simulink model "platafomra_esfera"  (R2018b)
settings: Solver=FixedStepAuto  StartTime=0.0  StopTime=30  FixedStep=0.001  RelTol=1e-4
model workspace: external: MATLAB File C:\Users\yomer\OneDrive\MATLAB\tesis\simulacion\platafomra_esfera_DataFile.m (data not in the file)
undefined symbols (not defined in the file or in its folder): a, B, b, HPrd, HPrn, HPtd, HPtn, LPd, LPn, P, rate_lim, smiData, X, Y, Z, z
libraries: sm_lib x73, nesl_utility x19, simulink x3
(part 3 of 3)

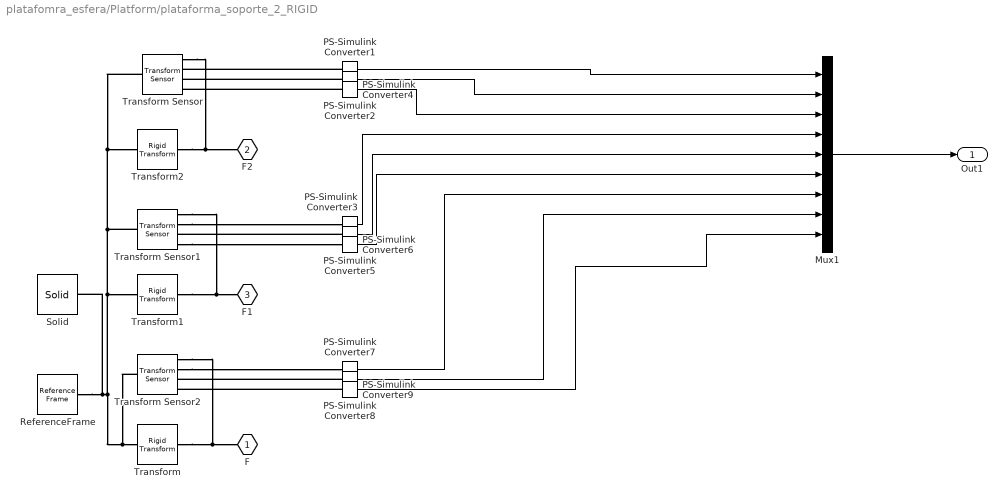
== system platafomra_esfera/Platform/plataforma_soporte_2_RIGID ==
  Mux1 : Mux  Inputs=9
  PS-Simulink Converter{1..9} (9 alike) : nesl_utility/PS-Simulink Converter  PhysicalDomain=network_engine_domain  SubClassName=ps_output  LeftPortType=input  RightPortType=output  PseudoPeriodic=off  Frequencies=[]  Unit=1  AffineConversion=off
  ReferenceFrame : sm_lib/Frames and Transforms/Reference Frame
  Solid : sm_lib/Body Elements/Solid  InertiaType=Custom  Mass=smiData.Solid(7).mass  MassUnits=kg  CenterOfMass=smiData.Solid(7).CoM  CenterOfMassUnits=mm  MomentsOfInertia=smiData.Solid(7).MoI  MomentsOfInertiaUnits=kg*mm^2  ProductsOfInertia=smiData.Solid(7).PoI  ProductsOfInertiaUnits=kg*mm^2  BasedOnType=Density  Density=1000  DensityUnits=kg/m^3  DoExposeReferenceFrame=on  SerializedFrames=<Frames/>  GraphicType=FromGeometry  MarkerShape=Sphere  MarkerSize=10  GraphicVisPropType=SimpleVisualProperties  GraphicDiffuseColor=smiData.Solid(7).color  GraphicSpecularColor=[0.5 0.5 0.5 1.0]  GraphicAmbientColor=[0.15 0.15 0.15 1.0]  GraphicEmissiveColor=[0.0 0.0 0.0 1.0]  GraphicShininess=75  GraphicOpacity=smiData.Solid(7).opacity  GeometryShape=FromFile  RectangleSize=[1 1]  RectangleSizeUnits=m  BrickDimensions=[1 1 1]  BrickDimensionUnits=m  CylinderRadius=1  CylinderRadiusUnits=m  CylinderLength=1  CylinderLengthUnits=m  SphereRadius=1  SphereRadiusUnits=m  EllipsoidRadii=[1 1 1]  EllipsoidRadiiUnits=m  ExtrusionCrossSection=[1 1; -1 1; -1 -1; 1 -1]  ExtrusionCrossSectionUnits=m  ExtrusionLength=1  ExtrusionLengthUnits=m  PolygonNumSides=3  PolygonOuterRadius=1  PolygonOuterRadiusUnits=m  ExtGeomFileType=STEP  ExtGeomFileName=plataforma_soporte_Predeterminado_sldprt.STEP  ExtGeomFileUnits=m  RevolutionCrossSection=[1 1; 1 -1; 2 -1; 2 1]  RevolutionCrossSectionUnits=m  RevolutionExtent=Full  RevolutionAngle=180  RevolutionAngleUnits=deg
  Transform : sm_lib/Frames and Transforms/Rigid Transform  TranslationMethod=Cartesian  TranslationStandardOffset=0  TranslationLengthUnit=mm  TranslationStandardAxis=+Z  TranslationCartesianOffset=smiData.RigidTransform(14).translation  TranslationROffset=0  TranslationROffsetUnits=m  TranslationZOffset=0  TranslationZOffsetUnits=m  TranslationThetaOffset=0  TranslationThetaOffsetUnits=deg  RotationMethod=ArbitraryAxis  RotationAngleUnits=rad  RotationStandardAxis=+Z  RotationAngle=smiData.RigidTransform(14).angle  RotationArbitraryAxis=smiData.RigidTransform(14).axis  FollAlignAxisA=+X  BaseAlignAxisA=+Y  FollAlignAxisB=+Y  BaseAlignAxisB=+Z  RotationSequenceAxes=FollowerAxes  RotationSequence=XYX  RotationSequenceAngles=[0 0 0]  RotationSequenceAnglesUnits=deg  RotationMatrix=[1 0 0; 0 1 0; 0 0 1]
  Transform Sensor : sm_lib/Frames and Transforms/Transform Sensor  MeasurementFrame=World  SenseAngle=off  SenseAxis=off  SenseAngle1=off  SenseAngle2=off  SenseAngle3=off  SenseQ=off  SenseR=off  SenseOmegaX=off  SenseOmegaY=off  SenseOmegaZ=off  SenseOmega1=off  SenseOmega2=off  SenseOmega3=off  SenseQDot=off  SenseRDot=off  SenseAlphaX=off  SenseAlphaY=off  SenseAlphaZ=off  SenseAlpha1=off  SenseAlpha2=off  SenseAlpha3=off  SenseQDDot=off  SenseRDDot=off  SenseX=on  SenseY=on  SenseZ=on  SenseRad=off  SenseAzim=off  SenseDist=off  SenseInc=off  SenseXDot=off  SenseYDot=off  SenseZDot=off  SenseRadDot=off  SenseAzimDot=off  SenseDistDot=off  SenseIncDot=off  SenseXDDot=off  SenseYDDot=off  SenseZDDot=off  SenseRadDDot=off  SenseAzimDDot=off  SenseDistDDot=off  SenseIncDDot=off
  Transform Sensor1 : sm_lib/Frames and Transforms/Transform Sensor  MeasurementFrame=World  SenseAngle=off  SenseAxis=off  SenseAngle1=off  SenseAngle2=off  SenseAngle3=off  SenseQ=off  SenseR=off  SenseOmegaX=off  SenseOmegaY=off  SenseOmegaZ=off  SenseOmega1=off  SenseOmega2=off  SenseOmega3=off  SenseQDot=off  SenseRDot=off  SenseAlphaX=off  SenseAlphaY=off  SenseAlphaZ=off  SenseAlpha1=off  SenseAlpha2=off  SenseAlpha3=off  SenseQDDot=off  SenseRDDot=off  SenseX=on  SenseY=on  SenseZ=on  SenseRad=off  SenseAzim=off  SenseDist=off  SenseInc=off  SenseXDot=off  SenseYDot=off  SenseZDot=off  SenseRadDot=off  SenseAzimDot=off  SenseDistDot=off  SenseIncDot=off  SenseXDDot=off  SenseYDDot=off  SenseZDDot=off  SenseRadDDot=off  SenseAzimDDot=off  SenseDistDDot=off  SenseIncDDot=off
  Transform Sensor2 : sm_lib/Frames and Transforms/Transform Sensor  MeasurementFrame=World  SenseAngle=off  SenseAxis=off  SenseAngle1=off  SenseAngle2=off  SenseAngle3=off  SenseQ=off  SenseR=off  SenseOmegaX=off  SenseOmegaY=off  SenseOmegaZ=off  SenseOmega1=off  SenseOmega2=off  SenseOmega3=off  SenseQDot=off  SenseRDot=off  SenseAlphaX=off  SenseAlphaY=off  SenseAlphaZ=off  SenseAlpha1=off  SenseAlpha2=off  SenseAlpha3=off  SenseQDDot=off  SenseRDDot=off  SenseX=on  SenseY=on  SenseZ=on  SenseRad=off  SenseAzim=off  SenseDist=off  SenseInc=off  SenseXDot=off  SenseYDot=off  SenseZDot=off  SenseRadDot=off  SenseAzimDot=off  SenseDistDot=off  SenseIncDot=off  SenseXDDot=off  SenseYDDot=off  SenseZDDot=off  SenseRadDDot=off  SenseAzimDDot=off  SenseDistDDot=off  SenseIncDDot=off
  Transform1 : sm_lib/Frames and Transforms/Rigid Transform  TranslationMethod=Cartesian  TranslationStandardOffset=0  TranslationLengthUnit=mm  TranslationStandardAxis=+Z  TranslationCartesianOffset=smiData.RigidTransform(16).translation  TranslationROffset=0  TranslationROffsetUnits=m  TranslationZOffset=0  TranslationZOffsetUnits=m  TranslationThetaOffset=0  TranslationThetaOffsetUnits=deg  RotationMethod=ArbitraryAxis  RotationAngleUnits=rad  RotationStandardAxis=+Z  RotationAngle=smiData.RigidTransform(16).angle  RotationArbitraryAxis=smiData.RigidTransform(16).axis  FollAlignAxisA=+X  BaseAlignAxisA=+Y  FollAlignAxisB=+Y  BaseAlignAxisB=+Z  RotationSequenceAxes=FollowerAxes  RotationSequence=XYX  RotationSequenceAngles=[0 0 0]  RotationSequenceAnglesUnits=deg  RotationMatrix=[1 0 0; 0 1 0; 0 0 1]
  Transform2 : sm_lib/Frames and Transforms/Rigid Transform  TranslationMethod=Cartesian  TranslationStandardOffset=0  TranslationLengthUnit=mm  TranslationStandardAxis=+Z  TranslationCartesianOffset=smiData.RigidTransform(18).translation  TranslationROffset=0  TranslationROffsetUnits=m  TranslationZOffset=0  TranslationZOffsetUnits=m  TranslationThetaOffset=0  TranslationThetaOffsetUnits=deg  RotationMethod=ArbitraryAxis  RotationAngleUnits=rad  RotationStandardAxis=+Z  RotationAngle=smiData.RigidTransform(18).angle  RotationArbitraryAxis=smiData.RigidTransform(18).axis  FollAlignAxisA=+X  BaseAlignAxisA=+Y  FollAlignAxisB=+Y  BaseAlignAxisB=+Z  RotationSequenceAxes=FollowerAxes  RotationSequence=XYX  RotationSequenceAngles=[0 0 0]  RotationSequenceAnglesUnits=deg  RotationMatrix=[1 0 0; 0 1 0; 0 0 1]
  F : PMIOPort  Side=Left
  F2 : PMIOPort  Port=2  Side=Left
  F1 : PMIOPort  Port=3  Side=Left
  Out1 : Outport
  wires:
  PS-Simulink Converter5/1 -> Mux1/5
  PS-Simulink Converter8/1 -> Mux1/8
  PS-Simulink Converter3/1 -> Mux1/4
  PS-Simulink Converter6/1 -> Mux1/6
  PS-Simulink Converter7/1 -> Mux1/7
  PS-Simulink Converter9/1 -> Mux1/9
  PS-Simulink Converter4/1 -> Mux1/3
  PS-Simulink Converter1/1 -> Mux1/1
  PS-Simulink Converter2/1 -> Mux1/2
  Mux1/1 -> Out1/1
  connections:
  Solid/RConn1 -- ReferenceFrame/RConn1 -- Transform1/LConn1 -- Transform Sensor/LConn1 -- Transform2/LConn1 -- Transform Sensor1/LConn1 -- Transform Sensor2/LConn1 -- Transform/LConn1
  Transform/RConn1 -- Transform Sensor2/RConn1 -- F/RConn1
  Transform1/RConn1 -- Transform Sensor1/RConn1 -- F1/RConn1
  Transform2/RConn1 -- Transform Sensor/RConn1 -- F2/RConn1
  PS-Simulink Converter1/LConn1 -- Transform Sensor/RConn2
  PS-Simulink Converter2/LConn1 -- Transform Sensor/RConn3
  PS-Simulink Converter4/LConn1 -- Transform Sensor/RConn4
  PS-Simulink Converter9/LConn1 -- Transform Sensor2/RConn4
  PS-Simulink Converter8/LConn1 -- Transform Sensor2/RConn3
  Transform Sensor2/RConn2 -- PS-Simulink Converter7/LConn1
  Transform Sensor1/RConn4 -- PS-Simulink Converter6/LConn1
  PS-Simulink Converter5/LConn1 -- Transform Sensor1/RConn3
  Transform Sensor1/RConn2 -- PS-Simulink Converter3/LConn1

== system platafomra_esfera/Platform/viela2_1_RIGID ==
  ReferenceFrame : sm_lib/Frames and Transforms/Reference Frame
  Solid : sm_lib/Body Elements/Solid  InertiaType=Custom  Mass=smiData.Solid(6).mass  MassUnits=kg  CenterOfMass=smiData.Solid(6).CoM  CenterOfMassUnits=mm  MomentsOfInertia=smiData.Solid(6).MoI  MomentsOfInertiaUnits=kg*mm^2  ProductsOfInertia=smiData.Solid(6).PoI  ProductsOfInertiaUnits=kg*mm^2  BasedOnType=Density  Density=1000  DensityUnits=kg/m^3  DoExposeReferenceFrame=on  SerializedFrames=<Frames/>  GraphicType=FromGeometry  MarkerShape=Sphere  MarkerSize=10  GraphicVisPropType=SimpleVisualProperties  GraphicDiffuseColor=smiData.Solid(6).color  GraphicSpecularColor=[0.5 0.5 0.5 1.0]  GraphicAmbientColor=[0.15 0.15 0.15 1.0]  GraphicEmissiveColor=[0.0 0.0 0.0 1.0]  GraphicShininess=75  GraphicOpacity=smiData.Solid(6).opacity  GeometryShape=FromFile  RectangleSize=[1 1]  RectangleSizeUnits=m  BrickDimensions=[1 1 1]  BrickDimensionUnits=m  CylinderRadius=1  CylinderRadiusUnits=m  CylinderLength=1  CylinderLengthUnits=m  SphereRadius=1  SphereRadiusUnits=m  EllipsoidRadii=[1 1 1]  EllipsoidRadiiUnits=m  ExtrusionCrossSection=[1 1; -1 1; -1 -1; 1 -1]  ExtrusionCrossSectionUnits=m  ExtrusionLength=1  ExtrusionLengthUnits=m  PolygonNumSides=3  PolygonOuterRadius=1  PolygonOuterRadiusUnits=m  ExtGeomFileType=STEP  ExtGeomFileName=viela2_Predeterminado_sldprt.STEP  ExtGeomFileUnits=m  RevolutionCrossSection=[1 1; 1 -1; 2 -1; 2 1]  RevolutionCrossSectionUnits=m  RevolutionExtent=Full  RevolutionAngle=180  RevolutionAngleUnits=deg
  Transform : sm_lib/Frames and Transforms/Rigid Transform  TranslationMethod=Cartesian  TranslationStandardOffset=0  TranslationLengthUnit=mm  TranslationStandardAxis=+Z  TranslationCartesianOffset=smiData.RigidTransform(1).translation  TranslationROffset=0  TranslationROffsetUnits=m  TranslationZOffset=0  TranslationZOffsetUnits=m  TranslationThetaOffset=0  TranslationThetaOffsetUnits=deg  RotationMethod=ArbitraryAxis  RotationAngleUnits=rad  RotationStandardAxis=+Z  RotationAngle=smiData.RigidTransform(1).angle  RotationArbitraryAxis=smiData.RigidTransform(1).axis  FollAlignAxisA=+X  BaseAlignAxisA=+Y  FollAlignAxisB=+Y  BaseAlignAxisB=+Z  RotationSequenceAxes=FollowerAxes  RotationSequence=XYX  RotationSequenceAngles=[0 0 0]  RotationSequenceAnglesUnits=deg  RotationMatrix=[1 0 0; 0 1 0; 0 0 1]
  Transform1 : sm_lib/Frames and Transforms/Rigid Transform  TranslationMethod=Cartesian  TranslationStandardOffset=0  TranslationLengthUnit=mm  TranslationStandardAxis=+Z  TranslationCartesianOffset=smiData.RigidTransform(4).translation  TranslationROffset=0  TranslationROffsetUnits=m  TranslationZOffset=0  TranslationZOffsetUnits=m  TranslationThetaOffset=0  TranslationThetaOffsetUnits=deg  RotationMethod=ArbitraryAxis  RotationAngleUnits=rad  RotationStandardAxis=+Z  RotationAngle=smiData.RigidTransform(4).angle  RotationArbitraryAxis=smiData.RigidTransform(4).axis  FollAlignAxisA=+X  BaseAlignAxisA=+Y  FollAlignAxisB=+Y  BaseAlignAxisB=+Z  RotationSequenceAxes=FollowerAxes  RotationSequence=XYX  RotationSequenceAngles=[0 0 0]  RotationSequenceAnglesUnits=deg  RotationMatrix=[1 0 0; 0 1 0; 0 0 1]
  Transform2 : sm_lib/Frames and Transforms/Rigid Transform  TranslationMethod=Cartesian  TranslationStandardOffset=0  TranslationLengthUnit=mm  TranslationStandardAxis=+Z  TranslationCartesianOffset=smiData.RigidTransform(5).translation  TranslationROffset=0  TranslationROffsetUnits=m  TranslationZOffset=0  TranslationZOffsetUnits=m  TranslationThetaOffset=0  TranslationThetaOffsetUnits=deg  RotationMethod=ArbitraryAxis  RotationAngleUnits=rad  RotationStandardAxis=+Z  RotationAngle=smiData.RigidTransform(5).angle  RotationArbitraryAxis=smiData.RigidTransform(5).axis  FollAlignAxisA=+X  BaseAlignAxisA=+Y  FollAlignAxisB=+Y  BaseAlignAxisB=+Z  RotationSequenceAxes=FollowerAxes  RotationSequence=XYX  RotationSequenceAngles=[0 0 0]  RotationSequenceAnglesUnits=deg  RotationMatrix=[1 0 0; 0 1 0; 0 0 1]
  F1 : PMIOPort  Side=Left
  F2 : PMIOPort  Port=2  Side=Right
  F : PMIOPort  Port=3  Side=Right
  connections:
  Solid/RConn1 -- ReferenceFrame/RConn1 -- Transform/LConn1 -- Transform1/LConn1 -- Transform2/LConn1
  Transform/RConn1 -- F/RConn1
  Transform1/RConn1 -- F1/RConn1
  Transform2/RConn1 -- F2/RConn1

== system platafomra_esfera/Platform/viela3_1_RIGID ==
  ReferenceFrame : sm_lib/Frames and Transforms/Reference Frame
  Solid : sm_lib/Body Elements/Solid  InertiaType=Custom  Mass=smiData.Solid(5).mass  MassUnits=kg  CenterOfMass=smiData.Solid(5).CoM  CenterOfMassUnits=mm  MomentsOfInertia=smiData.Solid(5).MoI  MomentsOfInertiaUnits=kg*mm^2  ProductsOfInertia=smiData.Solid(5).PoI  ProductsOfInertiaUnits=kg*mm^2  BasedOnType=Density  Density=1000  DensityUnits=kg/m^3  DoExposeReferenceFrame=on  SerializedFrames=<Frames/>  GraphicType=FromGeometry  MarkerShape=Sphere  MarkerSize=10  GraphicVisPropType=SimpleVisualProperties  GraphicDiffuseColor=smiData.Solid(5).color  GraphicSpecularColor=[0.5 0.5 0.5 1.0]  GraphicAmbientColor=[0.15 0.15 0.15 1.0]  GraphicEmissiveColor=[0.0 0.0 0.0 1.0]  GraphicShininess=75  GraphicOpacity=smiData.Solid(5).opacity  GeometryShape=FromFile  RectangleSize=[1 1]  RectangleSizeUnits=m  BrickDimensions=[1 1 1]  BrickDimensionUnits=m  CylinderRadius=1  CylinderRadiusUnits=m  CylinderLength=1  CylinderLengthUnits=m  SphereRadius=1  SphereRadiusUnits=m  EllipsoidRadii=[1 1 1]  EllipsoidRadiiUnits=m  ExtrusionCrossSection=[1 1; -1 1; -1 -1; 1 -1]  ExtrusionCrossSectionUnits=m  ExtrusionLength=1  ExtrusionLengthUnits=m  PolygonNumSides=3  PolygonOuterRadius=1  PolygonOuterRadiusUnits=m  ExtGeomFileType=STEP  ExtGeomFileName=viela3_Predeterminado_sldprt.STEP  ExtGeomFileUnits=m  RevolutionCrossSection=[1 1; 1 -1; 2 -1; 2 1]  RevolutionCrossSectionUnits=m  RevolutionExtent=Full  RevolutionAngle=180  RevolutionAngleUnits=deg
  Transform : sm_lib/Frames and Transforms/Rigid Transform  TranslationMethod=Cartesian  TranslationStandardOffset=0  TranslationLengthUnit=mm  TranslationStandardAxis=+Z  TranslationCartesianOffset=smiData.RigidTransform(7).translation  TranslationROffset=0  TranslationROffsetUnits=m  TranslationZOffset=0  TranslationZOffsetUnits=m  TranslationThetaOffset=0  TranslationThetaOffsetUnits=deg  RotationMethod=ArbitraryAxis  RotationAngleUnits=rad  RotationStandardAxis=+Z  RotationAngle=smiData.RigidTransform(7).angle  RotationArbitraryAxis=smiData.RigidTransform(7).axis  FollAlignAxisA=+X  BaseAlignAxisA=+Y  FollAlignAxisB=+Y  BaseAlignAxisB=+Z  RotationSequenceAxes=FollowerAxes  RotationSequence=XYX  RotationSequenceAngles=[0 0 0]  RotationSequenceAnglesUnits=deg  RotationMatrix=[1 0 0; 0 1 0; 0 0 1]
  Transform1 : sm_lib/Frames and Transforms/Rigid Transform  TranslationMethod=Cartesian  TranslationStandardOffset=0  TranslationLengthUnit=mm  TranslationStandardAxis=+Z  TranslationCartesianOffset=smiData.RigidTransform(10).translation  TranslationROffset=0  TranslationROffsetUnits=m  TranslationZOffset=0  TranslationZOffsetUnits=m  TranslationThetaOffset=0  TranslationThetaOffsetUnits=deg  RotationMethod=ArbitraryAxis  RotationAngleUnits=rad  RotationStandardAxis=+Z  RotationAngle=smiData.RigidTransform(10).angle  RotationArbitraryAxis=smiData.RigidTransform(10).axis  FollAlignAxisA=+X  BaseAlignAxisA=+Y  FollAlignAxisB=+Y  BaseAlignAxisB=+Z  RotationSequenceAxes=FollowerAxes  RotationSequence=XYX  RotationSequenceAngles=[0 0 0]  RotationSequenceAnglesUnits=deg  RotationMatrix=[1 0 0; 0 1 0; 0 0 1]
  Transform2 : sm_lib/Frames and Transforms/Rigid Transform  TranslationMethod=Cartesian  TranslationStandardOffset=0  TranslationLengthUnit=mm  TranslationStandardAxis=+Z  TranslationCartesianOffset=smiData.RigidTransform(11).translation  TranslationROffset=0  TranslationROffsetUnits=m  TranslationZOffset=0  TranslationZOffsetUnits=m  TranslationThetaOffset=0  TranslationThetaOffsetUnits=deg  RotationMethod=ArbitraryAxis  RotationAngleUnits=rad  RotationStandardAxis=+Z  RotationAngle=smiData.RigidTransform(11).angle  RotationArbitraryAxis=smiData.RigidTransform(11).axis  FollAlignAxisA=+X  BaseAlignAxisA=+Y  FollAlignAxisB=+Y  BaseAlignAxisB=+Z  RotationSequenceAxes=FollowerAxes  RotationSequence=XYX  RotationSequenceAngles=[0 0 0]  RotationSequenceAnglesUnits=deg  RotationMatrix=[1 0 0; 0 1 0; 0 0 1]
  F1 : PMIOPort  Side=Left
  F2 : PMIOPort  Port=2  Side=Right
  F : PMIOPort  Port=3  Side=Right
  connections:
  Solid/RConn1 -- ReferenceFrame/RConn1 -- Transform/LConn1 -- Transform1/LConn1 -- Transform2/LConn1
  Transform/RConn1 -- F/RConn1
  Transform1/RConn1 -- F1/RConn1
  Transform2/RConn1 -- F2/RConn1

== system platafomra_esfera/Platform/viela_1_RIGID ==
  ReferenceFrame : sm_lib/Frames and Transforms/Reference Frame
  Solid : sm_lib/Body Elements/Solid  InertiaType=Custom  Mass=smiData.Solid(3).mass  MassUnits=kg  CenterOfMass=smiData.Solid(3).CoM  CenterOfMassUnits=mm  MomentsOfInertia=smiData.Solid(3).MoI  MomentsOfInertiaUnits=kg*mm^2  ProductsOfInertia=smiData.Solid(3).PoI  ProductsOfInertiaUnits=kg*mm^2  BasedOnType=Density  Density=1000  DensityUnits=kg/m^3  DoExposeReferenceFrame=on  SerializedFrames=<Frames/>  GraphicType=FromGeometry  MarkerShape=Sphere  MarkerSize=10  GraphicVisPropType=SimpleVisualProperties  GraphicDiffuseColor=smiData.Solid(3).color  GraphicSpecularColor=[0.5 0.5 0.5 1.0]  GraphicAmbientColor=[0.15 0.15 0.15 1.0]  GraphicEmissiveColor=[0.0 0.0 0.0 1.0]  GraphicShininess=75  GraphicOpacity=smiData.Solid(3).opacity  GeometryShape=FromFile  RectangleSize=[1 1]  RectangleSizeUnits=m  BrickDimensions=[1 1 1]  BrickDimensionUnits=m  CylinderRadius=1  CylinderRadiusUnits=m  CylinderLength=1  CylinderLengthUnits=m  SphereRadius=1  SphereRadiusUnits=m  EllipsoidRadii=[1 1 1]  EllipsoidRadiiUnits=m  ExtrusionCrossSection=[1 1; -1 1; -1 -1; 1 -1]  ExtrusionCrossSectionUnits=m  ExtrusionLength=1  ExtrusionLengthUnits=m  PolygonNumSides=3  PolygonOuterRadius=1  PolygonOuterRadiusUnits=m  ExtGeomFileType=STEP  ExtGeomFileName=viela_Predeterminado_sldprt.STEP  ExtGeomFileUnits=m  RevolutionCrossSection=[1 1; 1 -1; 2 -1; 2 1]  RevolutionCrossSectionUnits=m  RevolutionExtent=Full  RevolutionAngle=180  RevolutionAngleUnits=deg
  Transform : sm_lib/Frames and Transforms/Rigid Transform  TranslationMethod=Cartesian  TranslationStandardOffset=0  TranslationLengthUnit=mm  TranslationStandardAxis=+Z  TranslationCartesianOffset=smiData.RigidTransform(25).translation  TranslationROffset=0  TranslationROffsetUnits=m  TranslationZOffset=0  TranslationZOffsetUnits=m  TranslationThetaOffset=0  TranslationThetaOffsetUnits=deg  RotationMethod=ArbitraryAxis  RotationAngleUnits=rad  RotationStandardAxis=+Z  RotationAngle=smiData.RigidTransform(25).angle  RotationArbitraryAxis=smiData.RigidTransform(25).axis  FollAlignAxisA=+X  BaseAlignAxisA=+Y  FollAlignAxisB=+Y  BaseAlignAxisB=+Z  RotationSequenceAxes=FollowerAxes  RotationSequence=XYX  RotationSequenceAngles=[0 0 0]  RotationSequenceAnglesUnits=deg  RotationMatrix=[1 0 0; 0 1 0; 0 0 1]
  Transform1 : sm_lib/Frames and Transforms/Rigid Transform  TranslationMethod=Cartesian  TranslationStandardOffset=0  TranslationLengthUnit=mm  TranslationStandardAxis=+Z  TranslationCartesianOffset=smiData.RigidTransform(28).translation  TranslationROffset=0  TranslationROffsetUnits=m  TranslationZOffset=0  TranslationZOffsetUnits=m  TranslationThetaOffset=0  TranslationThetaOffsetUnits=deg  RotationMethod=ArbitraryAxis  RotationAngleUnits=rad  RotationStandardAxis=+Z  RotationAngle=smiData.RigidTransform(28).angle  RotationArbitraryAxis=smiData.RigidTransform(28).axis  FollAlignAxisA=+X  BaseAlignAxisA=+Y  FollAlignAxisB=+Y  BaseAlignAxisB=+Z  RotationSequenceAxes=FollowerAxes  RotationSequence=XYX  RotationSequenceAngles=[0 0 0]  RotationSequenceAnglesUnits=deg  RotationMatrix=[1 0 0; 0 1 0; 0 0 1]
  Transform2 : sm_lib/Frames and Transforms/Rigid Transform  TranslationMethod=Cartesian  TranslationStandardOffset=0  TranslationLengthUnit=mm  TranslationStandardAxis=+Z  TranslationCartesianOffset=smiData.RigidTransform(29).translation  TranslationROffset=0  TranslationROffsetUnits=m  TranslationZOffset=0  TranslationZOffsetUnits=m  TranslationThetaOffset=0  TranslationThetaOffsetUnits=deg  RotationMethod=ArbitraryAxis  RotationAngleUnits=rad  RotationStandardAxis=+Z  RotationAngle=smiData.RigidTransform(29).angle  RotationArbitraryAxis=smiData.RigidTransform(29).axis  FollAlignAxisA=+X  BaseAlignAxisA=+Y  FollAlignAxisB=+Y  BaseAlignAxisB=+Z  RotationSequenceAxes=FollowerAxes  RotationSequence=XYX  RotationSequenceAngles=[0 0 0]  RotationSequenceAnglesUnits=deg  RotationMatrix=[1 0 0; 0 1 0; 0 0 1]
  F1 : PMIOPort  Side=Left
  F : PMIOPort  Port=2  Side=Right
  F2 : PMIOPort  Port=3  Side=Right
  connections:
  Solid/RConn1 -- ReferenceFrame/RConn1 -- Transform/LConn1 -- Transform1/LConn1 -- Transform2/LConn1
  Transform/RConn1 -- F/RConn1
  Transform1/RConn1 -- F1/RConn1
  Transform2/RConn1 -- F2/RConn1

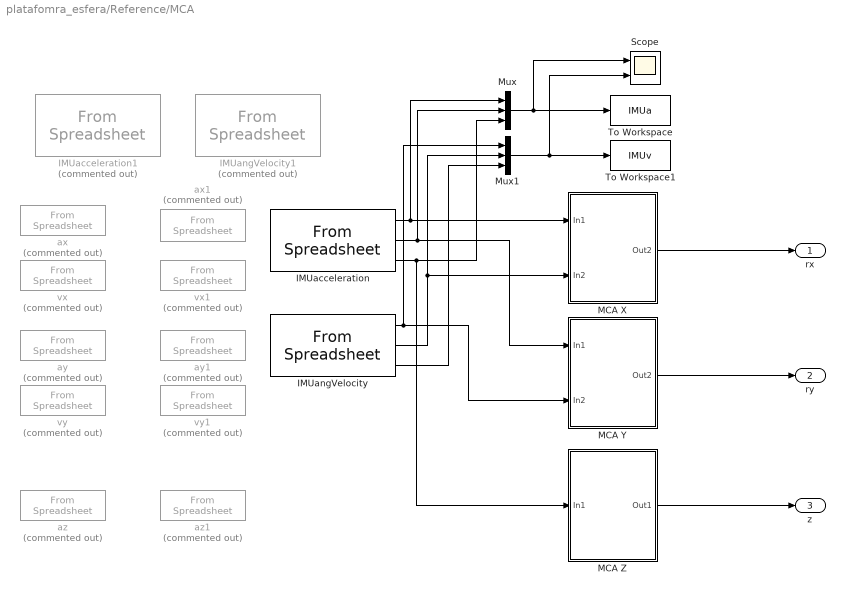
== system platafomra_esfera/Reference/MCA ==
  IMUacceleration : FromSpreadsheet  FileName=arrranqueparo2.xlsx  SheetName=Hoja1  Range=D2:F1014  TreatFirstColumnAs=Data  SampleTime=0.03
  IMUacceleration1 : FromSpreadsheet  Commented=on  FileName=vuelta90deg.xlsx  SheetName=Hoja1  Range=D2:F1089  TreatFirstColumnAs=Data  SampleTime=0.03
  IMUangVelocity : FromSpreadsheet  FileName=arrranqueparo2.xlsx  SheetName=Hoja1  Range=G2:I1014  TreatFirstColumnAs=Data  SampleTime=0.03
  IMUangVelocity1 : FromSpreadsheet  Commented=on  FileName=vuelta90deg.xlsx  SheetName=Hoja1  Range=G2:I1089  TreatFirstColumnAs=Data  SampleTime=0.03
  MCA X : Subsystem
  MCA Y : Subsystem
  MCA Z : Subsystem
  Mux : Mux  Inputs=3
  Mux1 : Mux  Inputs=3
  Scope : Scope  NumInputPorts=2
  To Workspace : ToWorkspace  VariableName=IMUa  SaveFormat=Timeseries  SampleTime=-1
  To Workspace1 : ToWorkspace  VariableName=IMUv  SaveFormat=Timeseries  SampleTime=-1
  ax : FromSpreadsheet  Commented=on  FileName=imu.xlsx  SheetName=Hoja1  Range=A1:A950  TreatFirstColumnAs=Data  SampleTime=0.016
  ax1 : FromSpreadsheet  Commented=on  FileName=arrranqueparo2.xlsx  SheetName=Hoja1  Range=D2:D1014  TreatFirstColumnAs=Data  SampleTime=0.03
  ay : FromSpreadsheet  Commented=on  FileName=imu.xlsx  SheetName=Hoja1  Range=B1:B950  TreatFirstColumnAs=Data  SampleTime=0.016
  ay1 : FromSpreadsheet  Commented=on  FileName=arrranqueparo.xlsx  SheetName=Hoja1  Range=B1:B1028  TreatFirstColumnAs=Data  SampleTime=0.016
  az : FromSpreadsheet  Commented=on  FileName=imu.xlsx  SheetName=Hoja1  Range=C1:C950  TreatFirstColumnAs=Data  SampleTime=0.016
  az1 : FromSpreadsheet  Commented=on  FileName=arrranqueparo.xlsx  SheetName=Hoja1  Range=C1:C1028  TreatFirstColumnAs=Data  SampleTime=0.016
  vx : FromSpreadsheet  Commented=on  FileName=imu.xlsx  SheetName=Hoja1  Range=D1:D950  TreatFirstColumnAs=Data  SampleTime=0.016
  vx1 : FromSpreadsheet  Commented=on  FileName=arrranqueparo.xlsx  SheetName=Hoja1  Range=D1:D1028  TreatFirstColumnAs=Data  SampleTime=0.016
  vy : FromSpreadsheet  Commented=on  FileName=imu.xlsx  SheetName=Hoja1  Range=E1:E950  TreatFirstColumnAs=Data  SampleTime=0.016
  vy1 : FromSpreadsheet  Commented=on  FileName=arrranqueparo.xlsx  SheetName=Hoja1  Range=E1:E1028  TreatFirstColumnAs=Data  SampleTime=0.016
  rx : Outport
  ry : Outport  Port=2
  z : Outport  Port=3
  wires:
  MCA Z/1(Out1) -> z/1
  Mux/1 -> Scope/1, To Workspace/1
  Mux1/1 -> Scope/2, To Workspace1/1
  MCA Y/1(Out2) -> ry/1
  MCA X/1(Out2) -> rx/1
  IMUacceleration/1 -> Mux/1, MCA X/1(In1)
  IMUacceleration/2 -> Mux/2, MCA Y/1(In1)
  IMUacceleration/3 -> Mux/3, MCA Z/1(In1)
  IMUangVelocity/1 -> MCA Y/2(In2), Mux1/1
  IMUangVelocity/2 -> MCA X/2(In2), Mux1/2
  IMUangVelocity/3 -> Mux1/3

== system platafomra_esfera/Reference/Subsystem1 ==
  t : Inport
  Add : Sum  Inputs=|++
  Add2 : Sum  Inputs=++|
  Sin : Trigonometry
  amp1 : Gain  Gain=5
  deg2rad : Gain  Gain=pi/180
  deg2rad2 : Gain  Gain=(pi/180)
  freq : Gain  Gain=360 * 3 / 10
  offset : Constant  Value=0  VectorParams1D=off
  phase : Constant  Value=0  VectorParams1D=off
  f : Outport
  wires:
  t/1 -> freq/1
  Add2/1 -> f/1
  offset/1 -> Add2/1
  freq/1 -> Add/1
  deg2rad/1 -> Sin/1
  Add/1 -> deg2rad/1
  amp1/1 -> deg2rad2/1
  Sin/1 -> amp1/1
  phase/1 -> Add/2
  deg2rad2/1 -> Add2/2

== system platafomra_esfera/Reference/Subsystem3 ==
  t : Inport
  Add : Sum  Inputs=|++
  Add2 : Sum  Inputs=++|
  Sin : Trigonometry
  amp1 : Gain  Gain=5
  deg2rad : Gain  Gain=pi/180
  deg2rad2 : Gain  Gain=(pi/180)
  freq : Gain  Gain=360 * 3 / 10
  offset : Constant  Value=0  VectorParams1D=off
  phase : Constant  Value=-90  VectorParams1D=off
  f : Outport
  wires:
  phase/1 -> Add/2
  Sin/1 -> amp1/1
  amp1/1 -> deg2rad2/1
  Add/1 -> deg2rad/1
  deg2rad/1 -> Sin/1
  freq/1 -> Add/1
  offset/1 -> Add2/1
  Add2/1 -> f/1
  t/1 -> freq/1
  deg2rad2/1 -> Add2/2

== system platafomra_esfera/Reference/Subsystem5 ==
  t : Inport
  Add : Sum  Inputs=|++
  Add2 : Sum  Inputs=++|
  Sin : Trigonometry
  amp1 : Gain  Gain=0.02
  deg2rad : Gain  Gain=pi/180
  freq : Gain  Gain=360 * 5/10
  offset : Constant  Value=0  VectorParams1D=off
  phase : Constant  Value=-90  VectorParams1D=off
  f : Outport
  wires:
  phase/1 -> Add/2
  Sin/1 -> amp1/1
  amp1/1 -> Add2/2
  Add/1 -> deg2rad/1
  deg2rad/1 -> Sin/1
  freq/1 -> Add/1
  offset/1 -> Add2/1
  Add2/1 -> f/1
  t/1 -> freq/1

== system platafomra_esfera/ADRC/Subsystem/ADRC ==
  note: V
  note: u
  x1 : Inport
  x2 : Inport  Port=2
  Z : Inport  Port=3
  xd : Inport  Port=4
  Demux : Demux  Outputs=2
  Derivative1 : Derivative
  MATLAB Function1 : MATLAB Function  TreatAsAtomicUnit=on
  Mux : Mux  Inputs=2
  Mux1 : Mux  Inputs=3
  Sum : Sum  Inputs=+-
  calculo de u : MATLAB Function  TreatAsAtomicUnit=on
  Out1 : Outport
  wires:
  Z/1 -> Sum/2
  calculo de u/1(u) -> Sum/1
  Sum/1 -> MATLAB Function1/1(u)
  MATLAB Function1/1(y) -> Out1/1
  x1/1 -> Mux/1
  x2/1 -> Mux/2
  Mux/1 -> calculo de u/1(x)
  Mux1/1 -> calculo de u/2(xd)
  Derivative1/1 -> Mux1/3
  xd/1 -> Demux/1
  Demux/1 -> Mux1/1
  Demux/2 -> Mux1/2, Derivative1/1

== system platafomra_esfera/ADRC/Subsystem/ADRC regulacion ==
  note: V
  note: u
  x1 : Inport
  x2 : Inport  Port=2
  Z : Inport  Port=3
  xd : Inport  Port=4
  Demux : Demux  Outputs=2
  MATLAB Function1 : MATLAB Function  TreatAsAtomicUnit=on
  Sum : Sum  Inputs=+-
  calculo de u : MATLAB Function  TreatAsAtomicUnit=on
  Out1 : Outport
  wires:
  x1/1 -> calculo de u/1(x1)
  Z/1 -> Sum/2
  calculo de u/1(u) -> Sum/1
  x2/1 -> calculo de u/2(x2)
  Sum/1 -> MATLAB Function1/1(u)
  MATLAB Function1/1(y) -> Out1/1
  xd/1 -> Demux/1
  Demux/1 -> calculo de u/3(xd)

== system platafomra_esfera/ADRC/Subsystem/Observador de Orden Extendido ==
  x1 : Inport
  v : Inport  Port=2
  Demux1 : Demux
  Integrator1 : Integrator  InitialCondition=[1.661;0;0;0]
  Observador : MATLAB Function  TreatAsAtomicUnit=on
  hatX1 : Outport
  hatX2 : Outport  Port=2
  z1 : Outport  Port=3
  wires:
  x1/1 -> Observador/2(x)
  Observador/1(dothatX) -> Integrator1/1
  v/1 -> Observador/3(u)
  Integrator1/1 -> Demux1/1, Observador/1(hatX)
  Demux1/1 -> hatX1/1
  Demux1/2 -> hatX2/1
  Demux1/3 -> z1/1

== system platafomra_esfera/ADRC/Subsystem/Planta ==
  note: ddq
  note: q
  note: dq
  z : Inport
  V : Inport  Port=2
  Integrator : Integrator
  Integrator1 : Integrator  InitialCondition=1.661
  MATLAB Function : MATLAB Function  TreatAsAtomicUnit=on
  Sum : Sum  Inputs=|+-
  q : Outport
  Out1 : Outport  Port=2
  wires:
  Integrator/1 -> Integrator1/1, MATLAB Function/2(dq)
  MATLAB Function/1(ddq) -> Sum/1
  Sum/1 -> Out1/1, Integrator/1
  Integrator1/1 -> q/1
  V/1 -> MATLAB Function/1(v)
  z/1 -> Sum/2

== system platafomra_esfera/ADRC/Subsystem/perturbacion ==
  Clock : Clock
  MATLAB Function : MATLAB Function  TreatAsAtomicUnit=on
  Out1 : Outport
  wires:
  MATLAB Function/1(y) -> Out1/1
  Clock/1 -> MATLAB Function/1(t)

== system platafomra_esfera/ADRC/Subsystem1/ADRC ==
  note: u
  note: V
  x1 : Inport
  x2 : Inport  Port=2
  Z : Inport  Port=3
  xd : Inport  Port=4
  Demux : Demux  Outputs=2
  Derivative1 : Derivative
  MATLAB Function1 : MATLAB Function  TreatAsAtomicUnit=on
  Mux : Mux  Inputs=2
  Mux1 : Mux  Inputs=3
  Sum : Sum  Inputs=+-
  calculo de u : MATLAB Function  TreatAsAtomicUnit=on
  Out1 : Outport
  wires:
  Demux/2 -> Derivative1/1, Mux1/2
  Demux/1 -> Mux1/1
  xd/1 -> Demux/1
  Derivative1/1 -> Mux1/3
  Mux1/1 -> calculo de u/2(xd)
  Mux/1 -> calculo de u/1(x)
  x2/1 -> Mux/2
  x1/1 -> Mux/1
  MATLAB Function1/1(y) -> Out1/1
  Sum/1 -> MATLAB Function1/1(u)
  calculo de u/1(u) -> Sum/1
  Z/1 -> Sum/2

== system platafomra_esfera/ADRC/Subsystem1/ADRC regulacion ==
  note: u
  note: V
  x1 : Inport
  x2 : Inport  Port=2
  Z : Inport  Port=3
  xd : Inport  Port=4
  Demux : Demux  Outputs=2
  MATLAB Function1 : MATLAB Function  TreatAsAtomicUnit=on
  Sum : Sum  Inputs=+-
  calculo de u : MATLAB Function  TreatAsAtomicUnit=on
  Out1 : Outport
  wires:
  Demux/1 -> calculo de u/3(xd)
  xd/1 -> Demux/1
  MATLAB Function1/1(y) -> Out1/1
  Sum/1 -> MATLAB Function1/1(u)
  x2/1 -> calculo de u/2(x2)
  calculo de u/1(u) -> Sum/1
  Z/1 -> Sum/2
  x1/1 -> calculo de u/1(x1)

== system platafomra_esfera/ADRC/Subsystem1/Observador de Orden Extendido ==
  x1 : Inport
  v : Inport  Port=2
  Demux1 : Demux
  Integrator1 : Integrator  InitialCondition=[-3.22;0;0;0]
  Observador : MATLAB Function  TreatAsAtomicUnit=on
  hatX1 : Outport
  hatX2 : Outport  Port=2
  z1 : Outport  Port=3
  wires:
  Demux1/3 -> z1/1
  Demux1/2 -> hatX2/1
  Demux1/1 -> hatX1/1
  Integrator1/1 -> Observador/1(hatX), Demux1/1
  v/1 -> Observador/3(u)
  Observador/1(dothatX) -> Integrator1/1
  x1/1 -> Observador/2(x)

== system platafomra_esfera/ADRC/Subsystem1/Planta ==
  note: dq
  note: q
  note: ddq
  z : Inport
  V : Inport  Port=2
  Integrator : Integrator
  Integrator1 : Integrator  InitialCondition=-3.22
  MATLAB Function : MATLAB Function  TreatAsAtomicUnit=on
  Sum : Sum  Inputs=|+-
  q : Outport
  Out1 : Outport  Port=2
  wires:
  z/1 -> Sum/2
  V/1 -> MATLAB Function/1(v)
  Integrator1/1 -> q/1
  Sum/1 -> Integrator/1, Out1/1
  MATLAB Function/1(ddq) -> Sum/1
  Integrator/1 -> MATLAB Function/2(dq), Integrator1/1

== system platafomra_esfera/ADRC/Subsystem1/perturbacion ==
  Clock : Clock
  MATLAB Function : MATLAB Function  TreatAsAtomicUnit=on
  Out1 : Outport
  wires:
  MATLAB Function/1(y) -> Out1/1
  Clock/1 -> MATLAB Function/1(t)

== system platafomra_esfera/ADRC/Subsystem2/ADRC ==
  note: V
  note: u
  x1 : Inport
  x2 : Inport  Port=2
  Z : Inport  Port=3
  xd : Inport  Port=4
  Demux : Demux  Outputs=2
  Derivative1 : Derivative
  MATLAB Function1 : MATLAB Function  TreatAsAtomicUnit=on
  Mux : Mux  Inputs=2
  Mux1 : Mux  Inputs=3
  Sum : Sum  Inputs=+-
  calculo de u : MATLAB Function  TreatAsAtomicUnit=on
  Out1 : Outport
  wires:
  Z/1 -> Sum/2
  calculo de u/1(u) -> Sum/1
  Sum/1 -> MATLAB Function1/1(u)
  MATLAB Function1/1(y) -> Out1/1
  x1/1 -> Mux/1
  x2/1 -> Mux/2
  Mux/1 -> calculo de u/1(x)
  Mux1/1 -> calculo de u/2(xd)
  Derivative1/1 -> Mux1/3
  xd/1 -> Demux/1
  Demux/1 -> Mux1/1
  Demux/2 -> Mux1/2, Derivative1/1

== system platafomra_esfera/ADRC/Subsystem2/ADRC regulacion ==
  note: V
  note: u
  x1 : Inport
  x2 : Inport  Port=2
  Z : Inport  Port=3
  xd : Inport  Port=4
  Demux : Demux  Outputs=2
  MATLAB Function1 : MATLAB Function  TreatAsAtomicUnit=on
  Sum : Sum  Inputs=+-
  calculo de u : MATLAB Function  TreatAsAtomicUnit=on
  Out1 : Outport
  wires:
  x1/1 -> calculo de u/1(x1)
  Z/1 -> Sum/2
  calculo de u/1(u) -> Sum/1
  x2/1 -> calculo de u/2(x2)
  Sum/1 -> MATLAB Function1/1(u)
  MATLAB Function1/1(y) -> Out1/1
  xd/1 -> Demux/1
  Demux/1 -> calculo de u/3(xd)

== system platafomra_esfera/ADRC/Subsystem2/Observador de Orden Extendido ==
  x1 : Inport
  v : Inport  Port=2
  Demux1 : Demux
  Integrator1 : Integrator  InitialCondition=[0.05;0;0;0]
  Observador : MATLAB Function  TreatAsAtomicUnit=on
  hatX1 : Outport
  hatX2 : Outport  Port=2
  z1 : Outport  Port=3
  wires:
  x1/1 -> Observador/2(x)
  Observador/1(dothatX) -> Integrator1/1
  v/1 -> Observador/3(u)
  Integrator1/1 -> Demux1/1, Observador/1(hatX)
  Demux1/1 -> hatX1/1
  Demux1/2 -> hatX2/1
  Demux1/3 -> z1/1

== system platafomra_esfera/ADRC/Subsystem2/Planta ==
  note: ddq
  note: q
  note: dq
  z : Inport
  V : Inport  Port=2
  Integrator : Integrator
  Integrator1 : Integrator  InitialCondition=0.05
  MATLAB Function : MATLAB Function  TreatAsAtomicUnit=on
  Sum : Sum  Inputs=|+-
  q : Outport
  Out1 : Outport  Port=2
  wires:
  Integrator/1 -> Integrator1/1, MATLAB Function/2(dq)
  MATLAB Function/1(ddq) -> Sum/1
  Sum/1 -> Out1/1, Integrator/1
  Integrator1/1 -> q/1
  V/1 -> MATLAB Function/1(v)
  z/1 -> Sum/2

== system platafomra_esfera/ADRC/Subsystem2/perturbacion ==
  Clock : Clock
  MATLAB Function : MATLAB Function  TreatAsAtomicUnit=on
  Out1 : Outport
  wires:
  MATLAB Function/1(y) -> Out1/1
  Clock/1 -> MATLAB Function/1(t)

== system platafomra_esfera/Inverse Kinematics/Pos Computation/6-Way Column Splitter ==
  A : Inport
  Column 1 : Selector  NumberOfDimensions=2  InputPortWidth=3  IndexOptions=Select all,Index vector (dialog)  Indices=-1,1  OutputSizes=1
  Column 2 : Selector  NumberOfDimensions=2  InputPortWidth=3  IndexOptions=Select all,Index vector (dialog)  Indices=-1,2  OutputSizes=1
  Column 3 : Selector  NumberOfDimensions=2  InputPortWidth=3  IndexOptions=Select all,Index vector (dialog)  Indices=-1,3  OutputSizes=1
  Col1 : Outport
  Col2 : Outport  Port=2
  Col3 : Outport  Port=3
  wires:
  A/1 -> Column 3/1, Column 2/1, Column 1/1
  Column 1/1 -> Col1/1
  Column 2/1 -> Col2/1
  Column 3/1 -> Col3/1

== system platafomra_esfera/Inverse Kinematics/Vel Computation/6-Way Column Splitter ==
  A : Inport
  Column 1 : Selector  NumberOfDimensions=2  InputPortWidth=3  IndexOptions=Select all,Index vector (dialog)  Indices=-1,1  OutputSizes=1
  Column 2 : Selector  NumberOfDimensions=2  InputPortWidth=3  IndexOptions=Select all,Index vector (dialog)  Indices=-1,2  OutputSizes=1
  Column 3 : Selector  NumberOfDimensions=2  InputPortWidth=3  IndexOptions=Select all,Index vector (dialog)  Indices=-1,3  OutputSizes=1
  Col1 : Outport
  Col2 : Outport  Port=2
  Col3 : Outport  Port=3
  wires:
  A/1 -> Column 3/1, Column 2/1, Column 1/1
  Column 1/1 -> Col1/1
  Column 2/1 -> Col2/1
  Column 3/1 -> Col3/1

== system platafomra_esfera/Reference/MCA/MCA X ==
  In1 : Inport
  In2 : Inport  Port=2
  Gain2 : Gain  Gain=0.5
  Gain3 : Gain  Gain=0.5
  HP rot : TransferFcn  Numerator=HPrn  Denominator=HPrd
  Integrator3 : Integrator
  LP tilt : TransferFcn  Numerator=LPn  Denominator=LPd
  Sum1 : Sum  Inputs=|++
  radtodeg : Gain  Commented=through  Gain=180/pi
  tilt coordination : Subsystem
  Out2 : Outport
  wires:
  In1/1 -> Gain2/1
  In2/1 -> Gain3/1
  Gain2/1 -> LP tilt/1
  Gain3/1 -> HP rot/1
  HP rot/1 -> Integrator3/1
  Integrator3/1 -> Sum1/2
  radtodeg/1 -> Out2/1
  Sum1/1 -> radtodeg/1
  LP tilt/1 -> tilt coordination/1(In1)
  tilt coordination/1(Out1) -> Sum1/1

== system platafomra_esfera/Reference/MCA/MCA Y ==
  In1 : Inport
  In2 : Inport  Port=2
  Gain2 : Gain  Gain=0.5
  Gain3 : Gain  Gain=0.5
  HP rot : TransferFcn  Numerator=HPrn  Denominator=HPrd
  Integrator3 : Integrator
  LP tilt : TransferFcn  Numerator=LPn  Denominator=LPd
  Sum1 : Sum  Inputs=|++
  radtodeg : Gain  Commented=through  Gain=180/pi
  tilt coordination : Subsystem
  Out2 : Outport
  wires:
  tilt coordination/1(Out1) -> Sum1/1
  LP tilt/1 -> tilt coordination/1(In1)
  Sum1/1 -> radtodeg/1
  radtodeg/1 -> Out2/1
  Integrator3/1 -> Sum1/2
  HP rot/1 -> Integrator3/1
  Gain3/1 -> HP rot/1
  Gain2/1 -> LP tilt/1
  In2/1 -> Gain3/1
  In1/1 -> Gain2/1

== system platafomra_esfera/Reference/MCA/MCA Z ==
  In1 : Inport
  Constant : Constant  Commented=on  Value=9.8
  Gain1 : Gain
  HP trans : TransferFcn  Numerator=HPtn  Denominator=HPtd
  Integrator1 : Integrator
  Integrator2 : Integrator
  Sum : Sum  Commented=on  Inputs=|+-
  radtodeg : Gain  Commented=through  Gain=180/pi
  Out1 : Outport
  wires:
  Gain1/1 -> HP trans/1
  HP trans/1 -> Integrator1/1
  Integrator1/1 -> Integrator2/1
  Integrator2/1 -> radtodeg/1
  radtodeg/1 -> Out1/1
  Constant/1 -> Sum/2
  In1/1 -> Gain1/1

== system platafomra_esfera/Reference/MCA/MCA X/tilt coordination ==
  In1 : Inport
  Gain : Gain  Gain=1/9.81
  Saturation : Saturate  UpperLimit=rate_lim*(pi/180)  LowerLimit=-rate_lim*(pi/180)  LinearizeAsGain=off
  Trigonometric Function : Trigonometry  Operator=atan
  Out1 : Outport
  wires:
  Trigonometric Function/1 -> Saturation/1
  In1/1 -> Gain/1
  Saturation/1 -> Out1/1
  Gain/1 -> Trigonometric Function/1

== system platafomra_esfera/Reference/MCA/MCA Y/tilt coordination ==
  In1 : Inport
  Gain : Gain  Gain=1/9.81
  Saturation : Saturate  UpperLimit=rate_lim*(pi/180)  LowerLimit=-rate_lim*(pi/180)  LinearizeAsGain=off
  Trigonometric Function : Trigonometry  Operator=atan
  Out1 : Outport
  wires:
  Gain/1 -> Trigonometric Function/1
  Saturation/1 -> Out1/1
  In1/1 -> Gain/1
  Trigonometric Function/1 -> Saturation/1

== matlab function platafomra_esfera/Inverse Kinematics/pos2rad M2/MATLAB Function ==
  data: L input; y output; z input; a input; b input
function y = fcn(L,z,a,b)

x=(a*a+L*L-b*b)/(2*a*L);
if x > 1
    x=1;
elseif x<-1
    x=-1;
end

w=z/L;
if w > 1
    w=1;
elseif w<-1
    w=-1;
end

alpha=acos(x);
beta=acos(w);
y = alpha+beta;

== matlab function platafomra_esfera/Inverse Kinematics/pos2rad M1/MATLAB Function ==
  data: L input; y output; z input; a input; b input
function y = fcn(L,z,a,b)

x=(a*a+L*L-b*b)/(2*a*L);
if x > 1
    x=1;
elseif x<-1
    x=-1;
end

w=z/L;
if w > 1
    w=1;
elseif w<-1
    w=-1;
end

alpha=acos(x);
beta=acos(w);
y = alpha+beta;

== matlab function platafomra_esfera/Inverse Kinematics/pos2rad M3/MATLAB Function ==
  data: L input; y output; z input; a input; b input
function y = fcn(L,z,a,b)

x=(a*a+L*L-b*b)/(2*a*L);
if x > 1
    x=1;
elseif x<-1
    x=-1;
end

w=z/L;
if w > 1
    w=1;
elseif w<-1
    w=-1;
end

alpha=acos(x);
beta=acos(w);
y = alpha+beta;

== matlab function platafomra_esfera/ADRC/Subsystem/ADRC/calculo de u ==
  data: x input; u output; xd input
function u = control(x,xd)
k1=10;
k2=20;

x1=x(1);
x2=x(2);
x1d=xd(1);
x2d=xd(2);
xdd=xd(3);
u = xdd-k1*(x1-x1d)-k2*(x2-x2d);

== matlab function platafomra_esfera/ADRC/Subsystem/ADRC/MATLAB Function1 ==
  data: u input; y output
function y = fcn(u)

R=6.14;
L=8.9e-3;
Jm=7.1e-6;
B=41e-6;
Kb=49.13e-3;
Ka=49.13e-3;
T=38e-3;
Vmax=24;
I=0.9;
P=14.3;
w=3600;
r=50;

y = u*((Jm*r*R)/Ka);

== matlab function platafomra_esfera/ADRC/Subsystem/Observador de Orden Extendido/Observador ==
  data: hatX input; x input; u input; dothatX output
function dothatX= ESO(hatX,x,u)

R=6.14;
L=8.9e-3;
Jm=7.1e-6;
B=41e-6;
Kb=49.13e-3;
Ka=49.13e-3;
T=38e-3;
Vmax=24;
I=0.9;
P=14.3;
w=3600;
r=50;

l0=40960000;
l1=2048000; 
l2=38400;
l3=320;

hatx1=hatX(1);
hatx2=hatX(2);
z1=hatX(3);
z2=hatX(4);

dothatx1=hatx2+l3*(x-hatx1);
dothatx2=u*(Ka/(Jm*r*R))+z1+l2*(x-hatx1);
dotz1=z2+l1*(x-hatx1);
dotz2=l0*(x-hatx1);
dothatX=[dothatx1;dothatx2;dotz1;dotz2];

== matlab function platafomra_esfera/ADRC/Subsystem/Planta/MATLAB Function ==
  data: v input; dq input; ddq output
function ddq  = fcn(v,dq)
R=6.14;
L=8.9e-3;
Jm=7.1e-6;
Bm=41e-6;
Kb=49.13e-3;
Ka=49.13e-3;
T=38e-3;
Vmax=24;
I=0.9;
P=14.3;
w=3600;
r=50;
JL=0.05;
BL=41e-6;
kL=0.99;
J=Jm+(JL/(r*r));
B=Bm+(BL/(r*r))+((Ka*Kb)/R);



% x1=-((B/J)*dq)-((kL/(J*r*r))*sin(q));
x1=-((Bm/Jm)+((Ka*Kb)/(Jm*R)))*dq;
x2=(Ka/(Jm*r*R));
ddq=x2*v+x1;

== matlab function platafomra_esfera/ADRC/Subsystem1/ADRC/MATLAB Function1 ==
  data: u input; y output
function y = fcn(u)

R=6.14;
L=8.9e-3;
Jm=7.1e-6;
B=41e-6;
Kb=49.13e-3;
Ka=49.13e-3;
T=38e-3;
Vmax=24;
I=0.9;
P=14.3;
w=3600;
r=50;

y = u*((Jm*r*R)/Ka);

== matlab function platafomra_esfera/ADRC/Subsystem1/ADRC/calculo de u ==
  data: x input; u output; xd input
function u = control(x,xd)
k1=10;
k2=20;

x1=x(1);
x2=x(2);
x1d=xd(1);
x2d=xd(2);
xdd=xd(3);
u = xdd-k1*(x1-x1d)-k2*(x2-x2d);

== matlab function platafomra_esfera/ADRC/Subsystem1/ADRC regulacion/MATLAB Function1 ==
  data: u input; y output
function y = fcn(u)

R=6.14;
L=8.9e-3;
Jm=7.1e-6;
B=41e-6;
Kb=49.13e-3;
Ka=49.13e-3;
T=38e-3;
Vmax=24;
I=0.9;
P=14.3;
w=3600;
r=5;

y = u*((Jm*r*R)/Ka);

== matlab function platafomra_esfera/ADRC/Subsystem1/ADRC regulacion/calculo de u ==
  data: x1 input; x2 input; u output; xd input
function u = control(x1,x2,xd)
k1=50;
k2=20;


u = -k1*(x1-xd)-k2*x2;

== matlab function platafomra_esfera/ADRC/Subsystem1/Observador de Orden Extendido/Observador ==
  data: hatX input; x input; u input; dothatX output
function dothatX= ESO(hatX,x,u)

R=6.14;
L=8.9e-3;
Jm=7.1e-6;
B=41e-6;
Kb=49.13e-3;
Ka=49.13e-3;
T=38e-3;
Vmax=24;
I=0.9;
P=14.3;
w=3600;
r=50;

l0=40960000;
l1=2048000; 
l2=38400;
l3=320;

hatx1=hatX(1);
hatx2=hatX(2);
z1=hatX(3);
z2=hatX(4);

dothatx1=hatx2+l3*(x-hatx1);
dothatx2=u*(Ka/(Jm*r*R))+z1+l2*(x-hatx1);
dotz1=z2+l1*(x-hatx1);
dotz2=l0*(x-hatx1);
dothatX=[dothatx1;dothatx2;dotz1;dotz2];

== matlab function platafomra_esfera/ADRC/Subsystem1/Planta/MATLAB Function ==
  data: v input; dq input; ddq output
function ddq  = fcn(v,dq)
R=6.14;
L=8.9e-3;
Jm=7.1e-6;
Bm=41e-6;
Kb=49.13e-3;
Ka=49.13e-3;
T=38e-3;
Vmax=24;
I=0.9;
P=14.3;
w=3600;
r=50;
JL=0.05;
BL=41e-6;
kL=0.99;
J=Jm+(JL/(r*r));
B=Bm+(BL/(r*r))+((Ka*Kb)/R);



% x1=-((B/J)*dq)-((kL/(J*r*r))*sin(q));
x1=-((Bm/Jm)+((Ka*Kb)/(Jm*R)))*dq;
x2=(Ka/(Jm*r*R));
ddq=x2*v+x1;

== matlab function platafomra_esfera/ADRC/Subsystem2/ADRC/MATLAB Function1 ==
  data: u input; y output
function y = fcn(u)

R=6.14;
L=8.9e-3;
Jm=7.1e-6;
B=41e-6;
Kb=49.13e-3;
Ka=49.13e-3;
T=38e-3;
Vmax=24;
I=0.9;
P=14.3;
w=3600;
r=50;

y = u*((Jm*r*R)/Ka);

== matlab function platafomra_esfera/ADRC/Subsystem2/ADRC/calculo de u ==
  data: x input; u output; xd input
function u = control(x,xd)
k1=10;
k2=20;

x1=x(1);
x2=x(2);
x1d=xd(1);
x2d=xd(2);
xdd=xd(3);
u = xdd-k1*(x1-x1d)-k2*(x2-x2d);

== matlab function platafomra_esfera/ADRC/Subsystem2/ADRC regulacion/MATLAB Function1 ==
  data: u input; y output
function y = fcn(u)

R=6.14;
L=8.9e-3;
Jm=7.1e-6;
B=41e-6;
Kb=49.13e-3;
Ka=49.13e-3;
T=38e-3;
Vmax=24;
I=0.9;
P=14.3;
w=3600;
r=5;

y = u*((Jm*r*R)/Ka);

== matlab function platafomra_esfera/ADRC/Subsystem2/ADRC regulacion/calculo de u ==
  data: x1 input; x2 input; u output; xd input
function u = control(x1,x2,xd)
k1=50;
k2=20;


u = -k1*(x1-xd)-k2*x2;

== matlab function platafomra_esfera/ADRC/Subsystem2/Observador de Orden Extendido/Observador ==
  data: hatX input; x input; u input; dothatX output
function dothatX= ESO(hatX,x,u)

R=6.14;
L=8.9e-3;
Jm=7.1e-6;
B=41e-6;
Kb=49.13e-3;
Ka=49.13e-3;
T=38e-3;
Vmax=24;
I=0.9;
P=14.3;
w=3600;
r=50;

l0=40960000;
l1=2048000; 
l2=38400;
l3=320;

hatx1=hatX(1);
hatx2=hatX(2);
z1=hatX(3);
z2=hatX(4);

dothatx1=hatx2+l3*(x-hatx1);
dothatx2=u*(Ka/(Jm*r*R))+z1+l2*(x-hatx1);
dotz1=z2+l1*(x-hatx1);
dotz2=l0*(x-hatx1);
dothatX=[dothatx1;dothatx2;dotz1;dotz2];

== matlab function platafomra_esfera/ADRC/Subsystem/ADRC regulacion/MATLAB Function1 ==
  data: u input; y output
function y = fcn(u)

R=6.14;
L=8.9e-3;
Jm=7.1e-6;
B=41e-6;
Kb=49.13e-3;
Ka=49.13e-3;
T=38e-3;
Vmax=24;
I=0.9;
P=14.3;
w=3600;
r=5;

y = u*((Jm*r*R)/Ka);

== matlab function platafomra_esfera/ADRC/Subsystem/ADRC regulacion/calculo de u ==
  data: x1 input; x2 input; u output; xd input
function u = control(x1,x2,xd)
k1=50;
k2=20;


u = -k1*(x1-xd)-k2*x2;

== matlab function platafomra_esfera/ADRC/Subsystem2/Planta/MATLAB Function ==
  data: v input; dq input; ddq output
function ddq  = fcn(v,dq)
R=6.14;
L=8.9e-3;
Jm=7.1e-6;
Bm=41e-6;
Kb=49.13e-3;
Ka=49.13e-3;
T=38e-3;
Vmax=24;
I=0.9;
P=14.3;
w=3600;
r=50;
JL=0.05;
BL=41e-6;
kL=0.99;
J=Jm+(JL/(r*r));
B=Bm+(BL/(r*r))+((Ka*Kb)/R);



% x1=-((B/J)*dq)-((kL/(J*r*r))*sin(q));
x1=-((Bm/Jm)+((Ka*Kb)/(Jm*R)))*dq;
x2=(Ka/(Jm*r*R));
ddq=x2*v+x1;

== matlab function platafomra_esfera/ADRC/Subsystem1/perturbacion/MATLAB Function ==
  data: t input; y output
function y = fcn(t)

y = 0.3+(2*exp(-(sin(20*t))^3))*((cos(30*t))^2);

== matlab function platafomra_esfera/ADRC/Subsystem/perturbacion/MATLAB Function ==
  data: t input; y output
function y = fcn(t)

y = 0.3+(2*exp(-(sin(20*t))^3))*((cos(30*t))^2);

== matlab function platafomra_esfera/ADRC/Subsystem2/perturbacion/MATLAB Function ==
  data: t input; y output
function y = fcn(t)

y = 0.3+(2*exp(-(sin(20*t))^3))*((cos(30*t))^2);

== matlab function platafomra_esfera/Inverse Kinematics/MATLAB Function ==
  data: pos input; y output; x input
function y  = fcn(pos,x)
u1=x(1);
u2=x(2);
if (pos(3) > 0.415)||(pos(3) < 0.271)
    u3=0;
else
    u3=x(3);
end
y = [u1,u2,u3];

== matlab function platafomra_esfera/Inverse Kinematics/MATLAB Function1 ==
  data: pos input; y output; x input
function y  = fcn(pos,x)
u1=x(1);
u2=x(2);
if (pos(3) > 0.410)||(pos(3) < 0.264)
    u3=0;
else
    u3=x(3);
end
y = [u1,u2,u3];

== matlab function platafomra_esfera/Inverse Kinematics/MATLAB Function2 ==
  data: pos input; y output; x input
function y  = fcn(pos,x)
u1=x(1);
u2=x(2);
if (pos(3) > 0.410)||(pos(3) < 0.264)
    u3=0;
else
    u3=x(3);
end
y = [u1,u2,u3];

== matlab function platafomra_esfera/Forward Kinematics/MATLAB Function ==
  data: x1 input; y output; x2 input; y1 input; y2 input; ref input
function y = fcn(x1,x2,y1,y2,ref)

m=(x2-x1)/(y2-y1);
x=ref+0.47;
b=y1-m*x1;

y = -m*0 + b;
